simulink model "reg_state_from_observer"  (R2014b)
settings: Solver=ode45  StartTime=0.0  StopTime=10.0  RelTol=1e-3
values from neighbouring files (symbols this model uses):
  A11 = A2(1,1)    [zad_10.m]
  A12 = A2(1,2:3)    [zad_10.m]
  A21 = A2(2:3,1)    [zad_10.m]
  A22 = A2(2:3,2:3)    [zad_10.m]
  B_1 = B2(1,1)    [zad_10.m]
  B_2 = B2(2:3,1)    [zad_10.m]
  x0 = [-1 -2 -3]    [zad_10.m]
  x0_observer = [ 0 0 ]    [zad_10.m]
undefined symbols (not defined in the file or in its folder): A2, B2, K, L, Tp
settings Model: Creator=Konrad  LastModifiedBy=Konrad

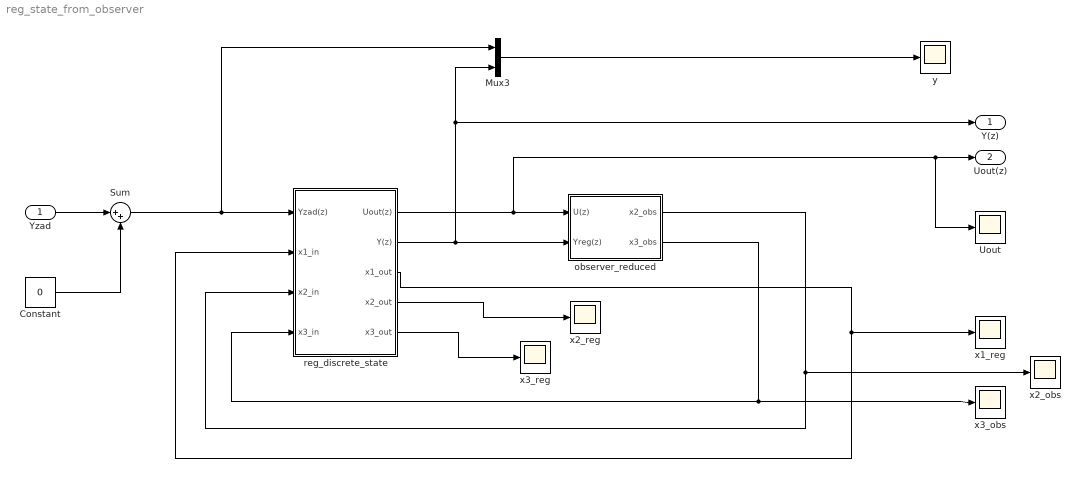
== system reg_state_from_observer ==
  Yzad : Inport
  Constant : Constant  Value=0
  Mux3 : Mux  Inputs=2
  Sum : Sum  Inputs=|++
  Uout : Scope
      settings: SaveName=ScopeData4
  observer_reduced : Subsystem
  reg_discrete_state : Subsystem
  x1_reg : Scope
  x2_obs : Scope
  x2_reg : Scope
      settings: SaveName=ScopeData5
  x3_obs : Scope
      settings: SaveName=ScopeData2
  x3_reg : Scope
      settings: SaveName=ScopeData6
  y : Scope
      settings: SaveName=ScopeData3
  Y(z) : Outport
  Uout(z) : Outport  Port=2
  wires:
  observer_reduced/1(x2_obs) -> reg_discrete_state/3(x2_in), x2_obs/1
  observer_reduced/2(x3_obs) -> x3_obs/1, reg_discrete_state/4(x3_in)
  Constant/1 -> Sum/2
  Yzad/1 -> Sum/1
  reg_discrete_state/1(Uout(z)) -> Uout/1, Uout(z)/1, observer_reduced/1(U(z))
  reg_discrete_state/2(Y(z)) -> observer_reduced/2(Yreg(z)), Mux3/2, Y(z)/1
  Sum/1 -> Mux3/1, reg_discrete_state/1(Yzad(z))
  Mux3/1 -> y/1
  reg_discrete_state/3(x1_out) -> x1_reg/1, reg_discrete_state/2("x1_in ")
  reg_discrete_state/4(x2_out) -> x2_reg/1
  reg_discrete_state/5(x3_out) -> x3_reg/1

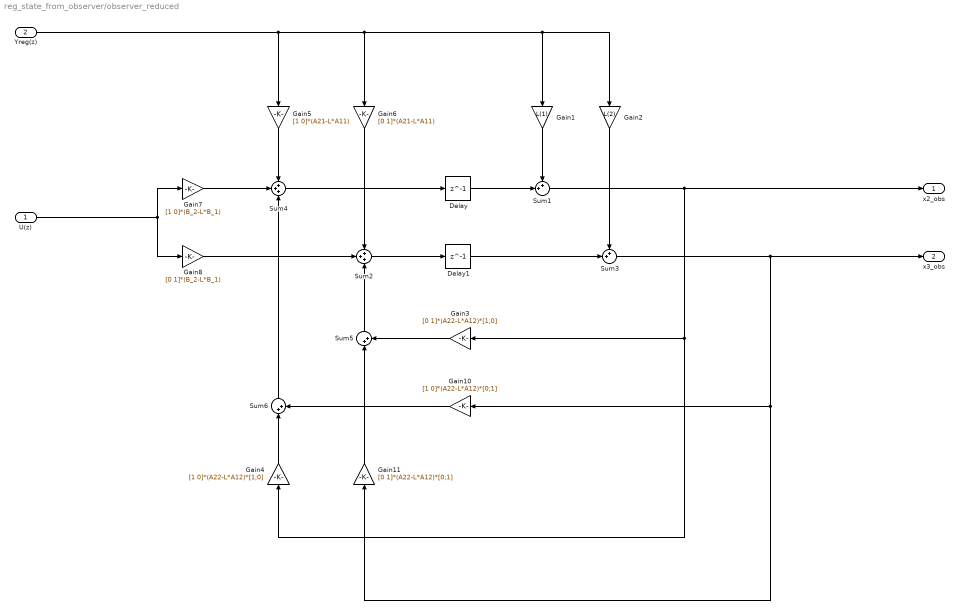
== system reg_state_from_observer/observer_reduced ==
  U(z) : Inport
  Yreg(z) : Inport  Port=2
  Delay : Delay  DelayLength=1  InitialCondition=x0_observer(1)  SampleTime=Tp
  Delay1 : Delay  DelayLength=1  InitialCondition=x0_observer(2)  SampleTime=Tp
  Gain1 : Gain  Gain=L(1)
  Gain10 : Gain  Gain=[1 0]*(A22-L*A12)*[0;1]
  Gain11 : Gain  Gain=[0 1]*(A22-L*A12)*[0;1]
  Gain2 : Gain  Gain=L(2)
  Gain3 : Gain  Gain=[0 1]*(A22-L*A12)*[1;0]
  Gain4 : Gain  Gain=[1 0]*(A22-L*A12)*[1;0]
  Gain5 : Gain  Gain=[1 0]*(A21-L*A11)
  Gain6 : Gain  Gain=[0 1]*(A21-L*A11)
  Gain7 : Gain  Gain=[1 0]*(B_2-L*B_1)
  Gain8 : Gain  Gain=[0 1]*(B_2-L*B_1)
  Sum1 : Sum  Inputs=++|
  Sum2 : Sum  Inputs=+++
  Sum3 : Sum  Inputs=++|
  Sum4 : Sum  Inputs=+++
  Sum5 : Sum  Inputs=|++
  Sum6 : Sum  Inputs=|++
  x2_obs : Outport
  x3_obs : Outport  Port=2
  wires:
  Gain4/1 -> Sum6/1
  U(z)/1 -> Gain7/1, Gain8/1
  Sum3/1 -> x3_obs/1, Gain11/1, Gain10/1
  Gain1/1 -> Sum1/1
  Delay/1 -> Sum1/2
  Gain5/1 -> Sum4/1
  Sum1/1 -> x2_obs/1, Gain4/1, Gain3/1
  Gain11/1 -> Sum5/1
  Gain7/1 -> Sum4/2
  Sum4/1 -> Delay/1
  Gain2/1 -> Sum3/1
  Sum6/1 -> Sum4/3
  Gain3/1 -> Sum5/2
  Delay1/1 -> Sum3/2
  Yreg(z)/1 -> Gain2/1, Gain1/1, Gain6/1, Gain5/1
  Gain10/1 -> Sum6/2
  Sum2/1 -> Delay1/1
  Gain8/1 -> Sum2/2
  Gain6/1 -> Sum2/1
  Sum5/1 -> Sum2/3

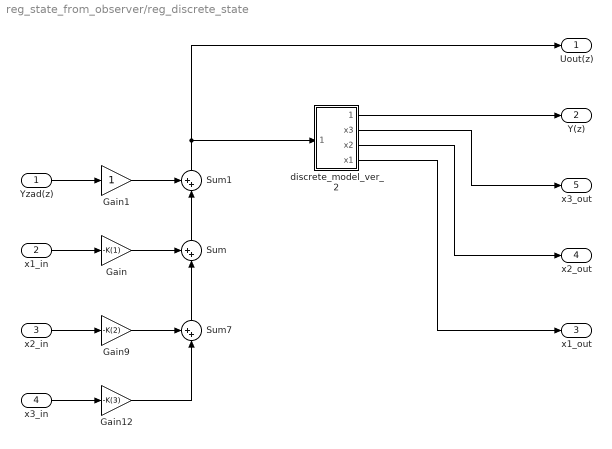
== system reg_state_from_observer/reg_discrete_state ==
  Yzad(z) : Inport
  "x1_in " : Inport  Port=2
  x2_in : Inport  Port=3
  x3_in : Inport  Port=4
  Gain : Gain  Gain=-K(1)
  Gain1 : Gain
  Gain12 : Gain  Gain=-K(3)
  Gain9 : Gain  Gain=-K(2)
  Sum : Sum  Inputs=++|
  Sum1 : Sum  Inputs=++|
  Sum7 : Sum  Inputs=++|
  discrete_model_ver_2 : Subsystem
  Uout(z) : Outport
  Y(z) : Outport  Port=2
  x1_out : Outport  Port=3
  x2_out : Outport  Port=4
  x3_out : Outport  Port=5
  wires:
  discrete_model_ver_2/1(Y(z)) -> Y(z)/1
  Gain9/1 -> Sum7/1
  discrete_model_ver_2/4(x1) -> x1_out/1
  discrete_model_ver_2/2(x3) -> x3_out/1
  Sum7/1 -> Sum/2
  discrete_model_ver_2/3(x2) -> x2_out/1
  Sum/1 -> Sum1/2
  Sum1/1 -> Uout(z)/1, discrete_model_ver_2/1(U(z))
  Gain1/1 -> Sum1/1
  Yzad(z)/1 -> Gain1/1
  Gain/1 -> Sum/1
  Gain12/1 -> Sum7/2
  x3_in/1 -> Gain12/1
  x2_in/1 -> Gain9/1
  "x1_in "/1 -> Gain/1

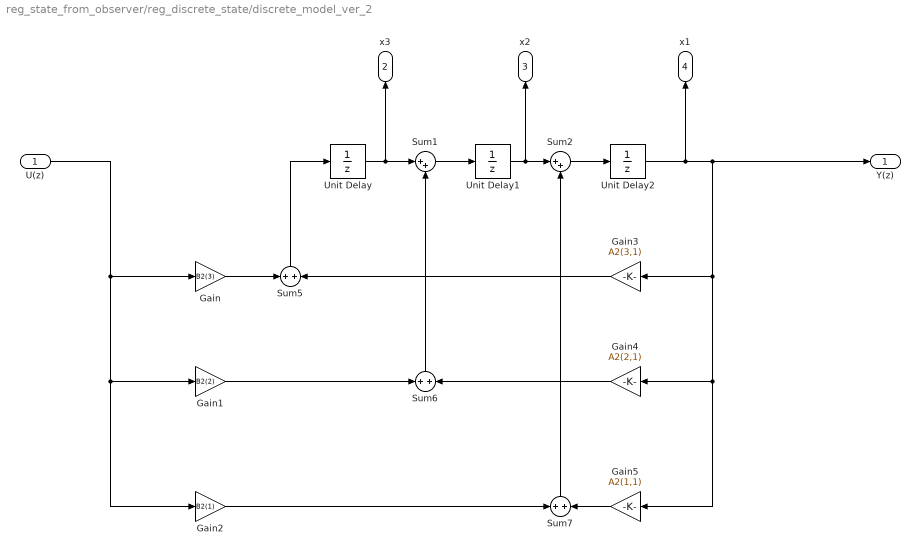
== system reg_state_from_observer/reg_discrete_state/discrete_model_ver_2 ==
  U(z) : Inport
  Gain : Gain  Gain=B2(3)
  Gain1 : Gain  Gain=B2(2)
  Gain2 : Gain  Gain=B2(1)
  Gain3 : Gain  Gain=A2(3,1)
  Gain4 : Gain  Gain=A2(2,1)
  Gain5 : Gain  Gain=A2(1,1)
  Sum1 : Sum  Inputs=|++
  Sum2 : Sum  Inputs=|++
  Sum5 : Sum  Inputs=+|+
  Sum6 : Sum  Inputs=+|+
  Sum7 : Sum  Inputs=+|+
  Unit Delay : UnitDelay  InitialCondition=x0(3)  SampleTime=Tp
  Unit Delay1 : UnitDelay  InitialCondition=x0(2)  SampleTime=Tp
  Unit Delay2 : UnitDelay  InitialCondition=x0(1)  SampleTime=Tp
  Y(z) : Outport
  x3 : Outport  Port=2
  x2 : Outport  Port=3
  x1 : Outport  Port=4
  wires:
  Sum1/1 -> Unit Delay1/1
  Unit Delay1/1 -> x2/1, Sum2/1
  Sum2/1 -> Unit Delay2/1
  Unit Delay/1 -> x3/1, Sum1/1
  Gain1/1 -> Sum6/1
  Gain4/1 -> Sum6/2
  Unit Delay2/1 -> x1/1, Y(z)/1, Gain3/1, Gain4/1, Gain5/1
  Gain3/1 -> Sum5/2
  Gain/1 -> Sum5/1
  Gain5/1 -> Sum7/2
  Sum7/1 -> Sum2/2
  Sum5/1 -> Unit Delay/1
  Gain2/1 -> Sum7/1
  Sum6/1 -> Sum1/2
  U(z)/1 -> Gain/1, Gain1/1, Gain2/1
